simulink model "chap3_2sim"  (Simulink 5.0)
settings: Solver=ode4  StartTime=0.0  StopTime=1.0  RelTol=1e-3
settings Model: LastModifiedBy=Administrator  ExtModeTrigMode=oneshot  ExtModeArmWhenConnect=off  SaveTime=off  SaveOutput=off  Decimation=100  LimitDataPoints=off  BooleanDataType=off

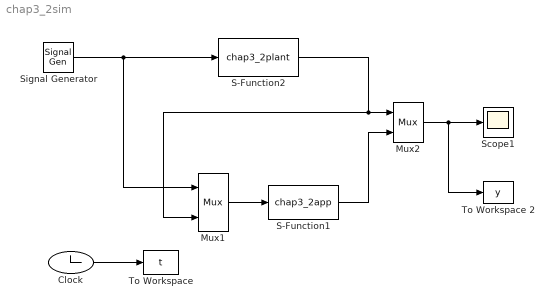
== system chap3_2sim ==
  Clock : Clock
  Mux1 : Mux  Inputs=2
  Mux2 : Mux  Inputs=2
  S-Function1 : S-Function  FunctionName=chap3_2app
  S-Function2 : S-Function  FunctionName=chap3_2plant
  Scope1 : Scope
      settings: TimeRange=0.2  YMin=-0.25  YMax=3  MaxDataPoints=50000  Decimation=0.001  SampleInput=on  SampleTime=0.001
  Signal Generator : SignalGenerator  Amplitude=0.5  Frequency=3
  To Workspace : ToWorkspace  VariableName=t  SampleTime=-1  SaveFormat=Array
  To Workspace 2 : ToWorkspace  VariableName=y  SampleTime=-1  SaveFormat=Array
  wires:
  Mux1/1 -> S-Function1/1
  S-Function2/1 -> Mux1/2, Mux2/1
  Signal Generator/1 -> S-Function2/1, Mux1/1
  S-Function1/1 -> Mux2/2
  Clock/1 -> To Workspace/1
  Mux2/1 -> Scope1/1, To Workspace 2/1
